simulink model "gazebodemo"  (R2022a)
settings: Solver=FixedStepAuto  StartTime=0.0  StopTime=10.0  FixedStep=0.001  RelTol=1e-3
values from neighbouring files (symbols this model uses):
  alpha = 10000    [Hopf_oscillator_sim.m]    (also in simulation_CPG.m)
  b = 100    [Hopf_oscillator_sim.m]    (also in simulation_CPG.m)
  f1 = 0    [Hopf_oscillator_sim.m]    (also in simulation_CPG.m)
  f2 = 0    [Hopf_oscillator_sim.m]    (also in simulation_CPG.m)
  K_d = diag([500,500])    [simulation_CPG.m]
  K_p = diag([500,500])    [simulation_CPG.m]
  lamda = 1    [Hopf_oscillator_sim.m]    (also in simulation_CPG.m)
  miu = 0.2    [Hopf_oscillator_sim.m]    (also in simulation_CPG.m)
  Tc = 0.001    [simulation_CPG.m]
  wst = (1-beta)/beta*wsw    (= 5.23598775598)    [Hopf_oscillator_sim.m]    (also in simulation_CPG.m)
  wsw = 5*pi    (= 15.7079632679)    [Hopf_oscillator_sim.m]    (also in simulation_CPG.m)
undefined symbols (not defined in the file or in its folder): a, effort, F_v, g, IFV, iner, joint_name, K, LF_body2thigh, LF_thigh2calf, LH_body2thigh, LH_thigh2calf, model_name, pi_m, RF_body2thigh, RF_thigh2calf, RH_body2thigh, RH_thigh2calf
libraries: robotgazebolib x26, simulink x16
settings Model: Creator=liltrump  LastModifiedBy=liltrump

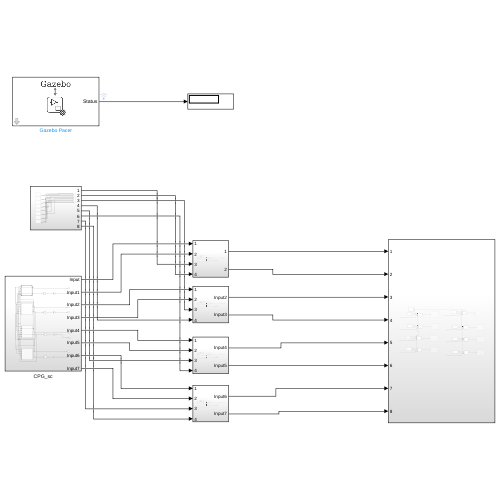
[thumbnail: Simulink's stored preview of the top-level diagram]
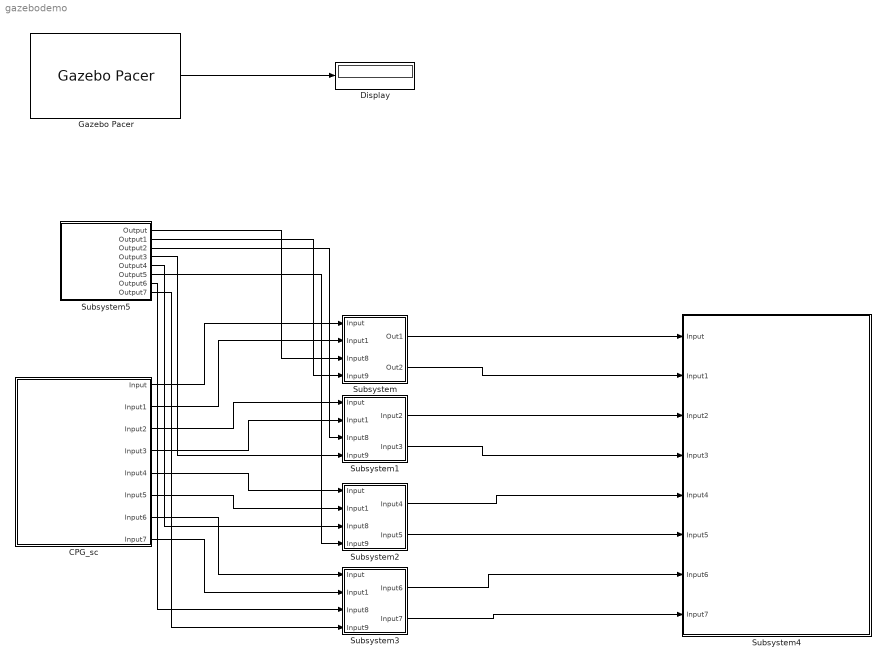
== system gazebodemo ==
  CPG_sc : Subsystem
  Display : Display
  Gazebo Pacer : robotgazebolib/Gazebo Pacer  ResetBehavior=Reset Gazebo simulation time  SampleTime=0.001
      settings: SourceProductBaseCode=RO
  Subsystem : Subsystem
  Subsystem1 : Subsystem
  Subsystem2 : Subsystem
  Subsystem3 : Subsystem
  Subsystem4 : Subsystem
  Subsystem5 : Subsystem
  wires:
  Gazebo Pacer/1 -> Display/1
  CPG_sc/1(Input) -> Subsystem/1(Input)
  CPG_sc/2(Input1) -> Subsystem/2(Input1)
  CPG_sc/3(Input2) -> Subsystem1/1(Input)
  CPG_sc/4(Input3) -> Subsystem1/2(Input1)
  CPG_sc/5(Input4) -> Subsystem2/1(Input)
  CPG_sc/8(Input7) -> Subsystem3/2(Input1)
  CPG_sc/6(Input5) -> Subsystem2/2(Input1)
  CPG_sc/7(Input6) -> Subsystem3/1(Input)
  Subsystem/1(Out1) -> Subsystem4/1(Input)
  Subsystem/2(Out2) -> Subsystem4/2(Input1)
  Subsystem1/1(Input2) -> Subsystem4/3(Input2)
  Subsystem1/2(Input3) -> Subsystem4/4(Input3)
  Subsystem2/1(Input4) -> Subsystem4/5(Input4)
  Subsystem2/2(Input5) -> Subsystem4/6(Input5)
  Subsystem3/1(Input6) -> Subsystem4/7(Input6)
  Subsystem3/2(Input7) -> Subsystem4/8(Input7)
  Subsystem5/1(Output) -> Subsystem/3(Input8)
  Subsystem5/2(Output1) -> Subsystem/4(Input9)
  Subsystem5/3(Output2) -> Subsystem1/3(Input8)
  Subsystem5/4(Output3) -> Subsystem1/4(Input9)
  Subsystem5/5(Output4) -> Subsystem2/3(Input8)
  Subsystem5/6(Output5) -> Subsystem2/4(Input9)
  Subsystem5/7(Output6) -> Subsystem3/3(Input8)
  Subsystem5/8(Output7) -> Subsystem3/4(Input9)

== system gazebodemo/CPG_sc ==
  Gain{,1..3} (4 alike) : Gain  Gain=-2
  Saturation{,1..3} (4 alike) : Saturate  UpperLimit=0  LowerLimit=-1
  Subsystem : Subsystem
  Subsystem1 : Subsystem
  Subsystem2 : Subsystem
  hopf1 : ModelReference  ModelNameDialog=Hopf.slx  SimulationMode=Normal  ModelReferenceVersion=1.13
  Input : Outport
  Input1 : Outport  Port=2
  Input2 : Outport  Port=3
  Input3 : Outport  Port=4
  Input4 : Outport  Port=5
  Input5 : Outport  Port=6
  Input6 : Outport  Port=7
  Input7 : Outport  Port=8
  wires:
  Saturation3/1 -> Gain3/1
  Subsystem2/2(Out2) -> Saturation3/1, Subsystem1/6(In6), Subsystem/6(In6), hopf1/6
  hopf1/1 -> Input/1, Subsystem2/1(In1), Subsystem1/1(In1), Subsystem/1(In1)
  hopf1/2 -> Saturation/1, Subsystem2/2(In2), Subsystem/2(In2), Subsystem1/2(In2)
  Subsystem1/2(Out2) -> Saturation2/1, Subsystem2/6(In6), Subsystem/4(In4), hopf1/4
  Saturation2/1 -> Gain2/1
  Gain/1 -> Input1/1
  Subsystem/2(Out2) -> Saturation1/1, Subsystem2/4(In4), Subsystem1/4(In4), hopf1/2
  Saturation/1 -> Gain/1
  Saturation1/1 -> Gain1/1
  Subsystem/1(Out1) -> Input2/1, Subsystem2/3(In3), Subsystem1/3(In3), hopf1/1
  Subsystem1/1(Out1) -> Input4/1, Subsystem/3(In3), hopf1/3, Subsystem2/5(In5)
  Gain2/1 -> Input5/1
  Subsystem2/1(Out1) -> Input6/1, Subsystem1/5(In5), Subsystem/5(In5), hopf1/5
  Gain1/1 -> Input3/1
  Gain3/1 -> Input7/1

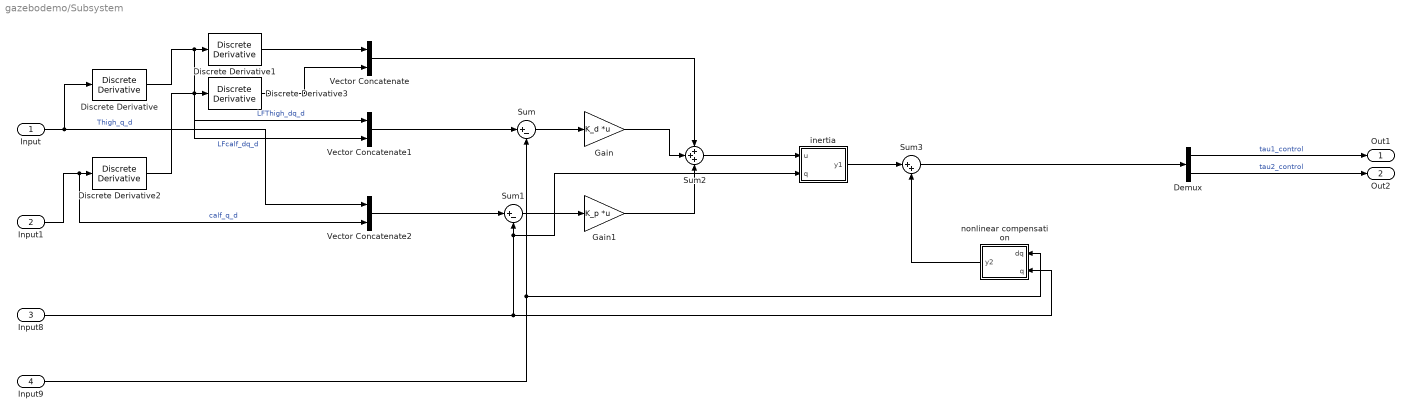
== system gazebodemo/Subsystem ==
  Input : Inport
  Input1 : Inport  Port=2
  Input8 : Inport  Port=3
  Input9 : Inport  Port=4
  Demux : Demux  Outputs=2
  Discrete Derivative{,1..3} (4 alike) : simulink/Discrete/Discrete Derivative  gainval=1.0  ICPrevScaledInput=0.0  OutMin=[]  OutMax=[]  OutDataType=fixdt(1, 16)  OutScaling=2^-10  DoSatur=off
  Gain : Gain  Gain=K_d  Multiplication=Matrix(K*u)
  Gain1 : Gain  Gain=K_p  Multiplication=Matrix(K*u)
  Sum : Sum  Inputs=|+-
  Sum1 : Sum  Inputs=|+-
  Sum2 : Sum  Inputs=+++
  Sum3 : Sum  Inputs=|++
  Vector Concatenate : Concatenate
  Vector Concatenate1 : Concatenate
  Vector Concatenate2 : Concatenate
  inertia : Subsystem
      mask Display: disp('B(q)u')
  nonlinear compensation : Subsystem
      mask Display: disp('n(q,dq)')
  Out1 : Outport
  Out2 : Outport  Port=2
  wires:
  Input/1 -> Vector Concatenate2/1, Discrete Derivative/1  "Thigh_q_d"
  Discrete Derivative/1 -> Vector Concatenate1/1, Discrete Derivative1/1  "LFThigh_dq_d"
  Input1/1 -> Vector Concatenate2/2, Discrete Derivative2/1  "calf_q_d"
  Discrete Derivative2/1 -> Vector Concatenate1/2, Discrete Derivative3/1  "LFcalf_dq_d"
  Gain1/1 -> Sum2/3
  Vector Concatenate1/1 -> Sum/1
  Sum3/1 -> Demux/1
  nonlinear compensation/1(y2) -> Sum3/2
  Vector Concatenate/1 -> Sum2/1
  inertia/1(y1) -> Sum3/1
  Sum/1 -> Gain/1
  Sum2/1 -> inertia/1(u)
  Sum1/1 -> Gain1/1
  Gain/1 -> Sum2/2
  Vector Concatenate2/1 -> Sum1/1
  Discrete Derivative1/1 -> Vector Concatenate/1
  Discrete Derivative3/1 -> Vector Concatenate/2
  Input8/1 -> nonlinear compensation/2(q), inertia/2(q), Sum1/2
  Input9/1 -> Sum/2, nonlinear compensation/1(dq)
  Demux/2 -> Out2/1  "tau2_control"
  Demux/1 -> Out1/1  "tau1_control"

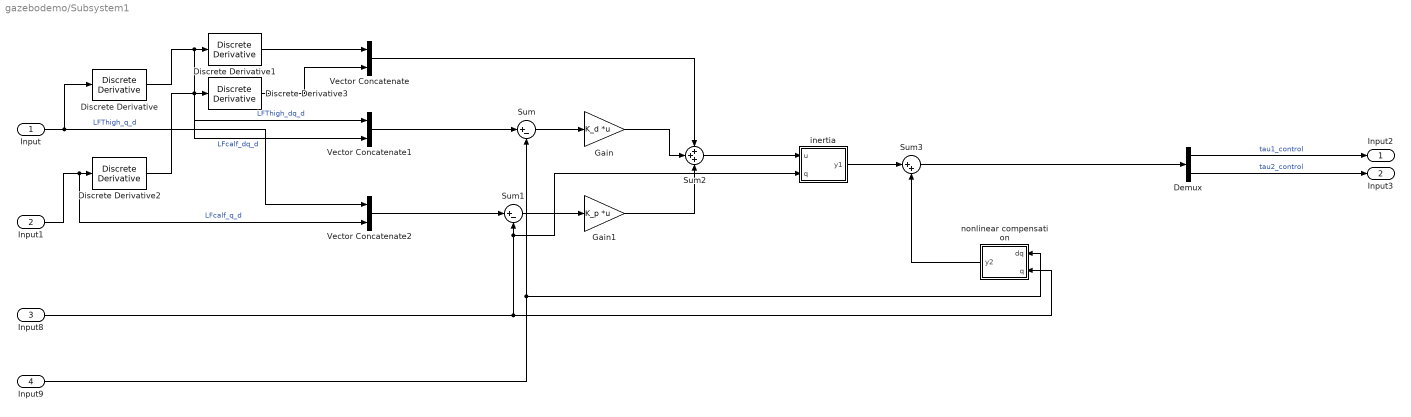
== system gazebodemo/Subsystem1 ==
  Input : Inport
  Input1 : Inport  Port=2
  Input8 : Inport  Port=3
  Input9 : Inport  Port=4
  Demux : Demux  Outputs=2
  Discrete Derivative{,1..3} (4 alike) : simulink/Discrete/Discrete Derivative  gainval=1.0  ICPrevScaledInput=0.0  OutMin=[]  OutMax=[]  OutDataType=fixdt(1, 16)  OutScaling=2^-10  DoSatur=off
  Gain : Gain  Gain=K_d  Multiplication=Matrix(K*u)
  Gain1 : Gain  Gain=K_p  Multiplication=Matrix(K*u)
  Sum : Sum  Inputs=|+-
  Sum1 : Sum  Inputs=|+-
  Sum2 : Sum  Inputs=+++
  Sum3 : Sum  Inputs=|++
  Vector Concatenate : Concatenate
  Vector Concatenate1 : Concatenate
  Vector Concatenate2 : Concatenate
  inertia : Subsystem
      mask Display: disp('B(q)u')
  nonlinear compensation : Subsystem
      mask Display: disp('n(q,dq)')
  Input2 : Outport
  Input3 : Outport  Port=2
  wires:
  Input/1 -> Vector Concatenate2/1, Discrete Derivative/1  "LFThigh_q_d"
  Discrete Derivative/1 -> Vector Concatenate1/1, Discrete Derivative1/1  "LFThigh_dq_d"
  Input1/1 -> Vector Concatenate2/2, Discrete Derivative2/1  "LFcalf_q_d"
  Discrete Derivative2/1 -> Vector Concatenate1/2, Discrete Derivative3/1  "LFcalf_dq_d"
  Gain1/1 -> Sum2/3
  Vector Concatenate1/1 -> Sum/1
  Sum3/1 -> Demux/1
  nonlinear compensation/1(y2) -> Sum3/2
  Vector Concatenate/1 -> Sum2/1
  inertia/1(y1) -> Sum3/1
  Sum/1 -> Gain/1
  Sum2/1 -> inertia/1(u)
  Sum1/1 -> Gain1/1
  Gain/1 -> Sum2/2
  Vector Concatenate2/1 -> Sum1/1
  Discrete Derivative1/1 -> Vector Concatenate/1
  Discrete Derivative3/1 -> Vector Concatenate/2
  Input8/1 -> nonlinear compensation/2(q), inertia/2(q), Sum1/2
  Input9/1 -> Sum/2, nonlinear compensation/1(dq)
  Demux/2 -> Input3/1  "tau2_control"
  Demux/1 -> Input2/1  "tau1_control"

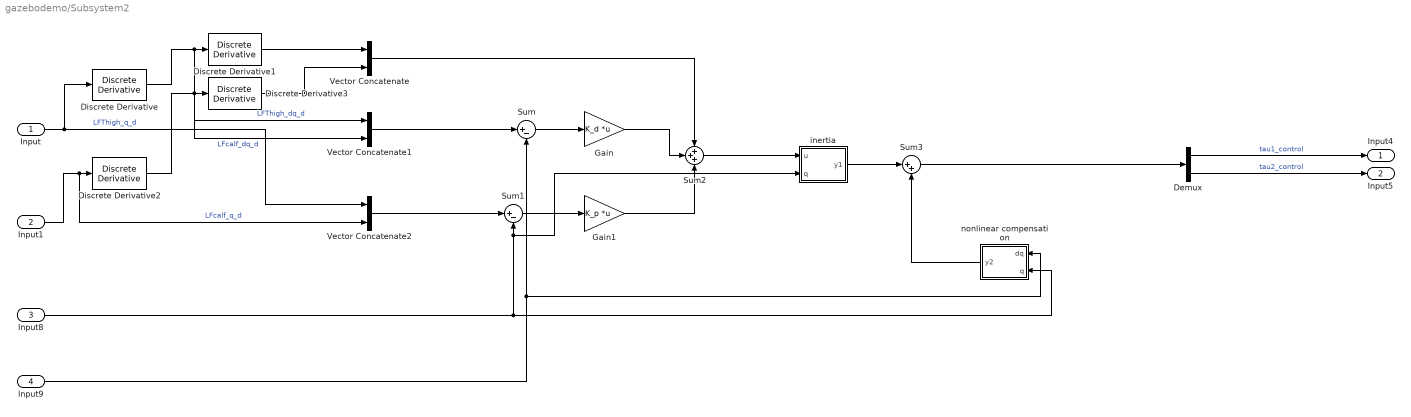
== system gazebodemo/Subsystem2 ==
  Input : Inport
  Input1 : Inport  Port=2
  Input8 : Inport  Port=3
  Input9 : Inport  Port=4
  Demux : Demux  Outputs=2
  Discrete Derivative{,1..3} (4 alike) : simulink/Discrete/Discrete Derivative  gainval=1.0  ICPrevScaledInput=0.0  OutMin=[]  OutMax=[]  OutDataType=fixdt(1, 16)  OutScaling=2^-10  DoSatur=off
  Gain : Gain  Gain=K_d  Multiplication=Matrix(K*u)
  Gain1 : Gain  Gain=K_p  Multiplication=Matrix(K*u)
  Sum : Sum  Inputs=|+-
  Sum1 : Sum  Inputs=|+-
  Sum2 : Sum  Inputs=+++
  Sum3 : Sum  Inputs=|++
  Vector Concatenate : Concatenate
  Vector Concatenate1 : Concatenate
  Vector Concatenate2 : Concatenate
  inertia : Subsystem
      mask Display: disp('B(q)u')
  nonlinear compensation : Subsystem
      mask Display: disp('n(q,dq)')
  Input4 : Outport
  Input5 : Outport  Port=2
  wires:
  Input/1 -> Vector Concatenate2/1, Discrete Derivative/1  "LFThigh_q_d"
  Discrete Derivative/1 -> Vector Concatenate1/1, Discrete Derivative1/1  "LFThigh_dq_d"
  Input1/1 -> Vector Concatenate2/2, Discrete Derivative2/1  "LFcalf_q_d"
  Discrete Derivative2/1 -> Vector Concatenate1/2, Discrete Derivative3/1  "LFcalf_dq_d"
  Gain1/1 -> Sum2/3
  Vector Concatenate1/1 -> Sum/1
  Sum3/1 -> Demux/1
  nonlinear compensation/1(y2) -> Sum3/2
  Vector Concatenate/1 -> Sum2/1
  inertia/1(y1) -> Sum3/1
  Sum/1 -> Gain/1
  Sum2/1 -> inertia/1(u)
  Sum1/1 -> Gain1/1
  Gain/1 -> Sum2/2
  Vector Concatenate2/1 -> Sum1/1
  Discrete Derivative1/1 -> Vector Concatenate/1
  Discrete Derivative3/1 -> Vector Concatenate/2
  Input8/1 -> nonlinear compensation/2(q), inertia/2(q), Sum1/2
  Input9/1 -> Sum/2, nonlinear compensation/1(dq)
  Demux/2 -> Input5/1  "tau2_control"
  Demux/1 -> Input4/1  "tau1_control"

== system gazebodemo/Subsystem3 ==
  Input : Inport
  Input1 : Inport  Port=2
  Input8 : Inport  Port=3
  Input9 : Inport  Port=4
  Demux : Demux  Outputs=2
  Discrete Derivative{,1..3} (4 alike) : simulink/Discrete/Discrete Derivative  gainval=1.0  ICPrevScaledInput=0.0  OutMin=[]  OutMax=[]  OutDataType=fixdt(1, 16)  OutScaling=2^-10  DoSatur=off
  Gain : Gain  Gain=K_d  Multiplication=Matrix(K*u)
  Gain1 : Gain  Gain=K_p  Multiplication=Matrix(K*u)
  Sum : Sum  Inputs=|+-
  Sum1 : Sum  Inputs=|+-
  Sum2 : Sum  Inputs=+++
  Sum3 : Sum  Inputs=|++
  Vector Concatenate : Concatenate
  Vector Concatenate1 : Concatenate
  Vector Concatenate2 : Concatenate
  inertia : Subsystem
      mask Display: disp('B(q)u')
  nonlinear compensation : Subsystem
      mask Display: disp('n(q,dq)')
  Input6 : Outport
  Input7 : Outport  Port=2
  wires:
  Input/1 -> Vector Concatenate2/1, Discrete Derivative/1  "LFThigh_q_d"
  Discrete Derivative/1 -> Vector Concatenate1/1, Discrete Derivative1/1  "LFThigh_dq_d"
  Input1/1 -> Vector Concatenate2/2, Discrete Derivative2/1  "LFcalf_q_d"
  Discrete Derivative2/1 -> Vector Concatenate1/2, Discrete Derivative3/1  "LFcalf_dq_d"
  Gain1/1 -> Sum2/3
  Vector Concatenate1/1 -> Sum/1
  Sum3/1 -> Demux/1
  nonlinear compensation/1(y2) -> Sum3/2
  Vector Concatenate/1 -> Sum2/1
  inertia/1(y1) -> Sum3/1
  Sum/1 -> Gain/1
  Sum2/1 -> inertia/1(u)
  Sum1/1 -> Gain1/1
  Gain/1 -> Sum2/2
  Vector Concatenate2/1 -> Sum1/1
  Discrete Derivative1/1 -> Vector Concatenate/1
  Discrete Derivative3/1 -> Vector Concatenate/2
  Input8/1 -> nonlinear compensation/2(q), inertia/2(q), Sum1/2
  Input9/1 -> Sum/2, nonlinear compensation/1(dq)
  Demux/2 -> Input7/1  "tau2_control"
  Demux/1 -> Input6/1  "tau1_control"

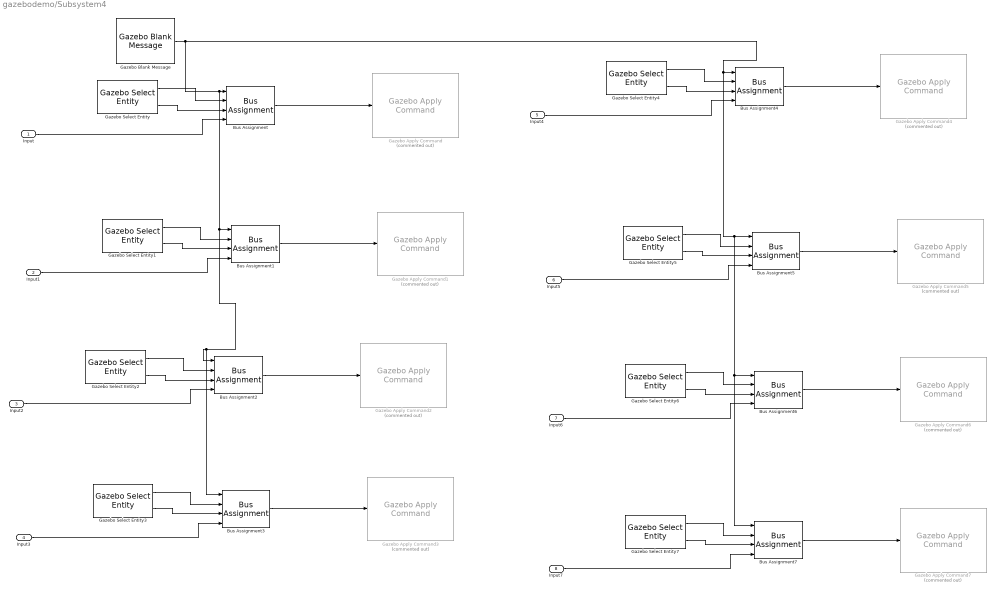
== system gazebodemo/Subsystem4 ==
  Input : Inport
  Input1 : Inport  Port=2
  Input2 : Inport  Port=3
  Input3 : Inport  Port=4
  Input4 : Inport  Port=5
  Input5 : Inport  Port=6
  Input6 : Inport  Port=7
  Input7 : Inport  Port=8
  Bus Assignment{,1..7} (8 alike) : BusAssignment  AssignedSignals=model_name,joint_name,effort
  Gazebo Apply Command{,1..7} (8 alike) : robotgazebolib/Gazebo Apply Command  Commented=on  cmdType=ApplyJointTorque  sampleTime=0.001
      settings: SourceProductBaseCode=RO
  Gazebo Blank Message : robotgazebolib/Gazebo Blank Message  msgType=ApplyJointTorque  sampleTime=0.001  busName='Gazebo_SL_Bus_gazebo_msgs_ApplyJointTorque'
      settings: SourceProductBaseCode=RO
  Gazebo Select Entity : robotgazebolib/Gazebo Select Entity  modelElemName=IFV/LF_body2thigh  outputArraySize=128  OutputLabel=Joint  SelectType=Joint
      settings: SourceProductBaseCode=RO
  Gazebo Select Entity1 : robotgazebolib/Gazebo Select Entity  modelElemName=IFV/LF_thigh2calf  outputArraySize=128  OutputLabel=Joint  SelectType=Joint
      settings: SourceProductBaseCode=RO
  Gazebo Select Entity2 : robotgazebolib/Gazebo Select Entity  modelElemName=IFV/RF_body2thigh  outputArraySize=128  OutputLabel=Joint  SelectType=Joint
      settings: SourceProductBaseCode=RO
  Gazebo Select Entity3 : robotgazebolib/Gazebo Select Entity  modelElemName=IFV/RF_thigh2calf  outputArraySize=128  OutputLabel=Joint  SelectType=Joint
      settings: SourceProductBaseCode=RO
  Gazebo Select Entity4 : robotgazebolib/Gazebo Select Entity  modelElemName=IFV/LH_body2thigh  outputArraySize=128  OutputLabel=Joint  SelectType=Joint
      settings: SourceProductBaseCode=RO
  Gazebo Select Entity5 : robotgazebolib/Gazebo Select Entity  modelElemName=IFV/LH_thigh2calf  outputArraySize=128  OutputLabel=Joint  SelectType=Joint
      settings: SourceProductBaseCode=RO
  Gazebo Select Entity6 : robotgazebolib/Gazebo Select Entity  modelElemName=IFV/RH_body2thigh  outputArraySize=128  OutputLabel=Joint  SelectType=Joint
      settings: SourceProductBaseCode=RO
  Gazebo Select Entity7 : robotgazebolib/Gazebo Select Entity  modelElemName=IFV/RH_thigh2calf  outputArraySize=128  OutputLabel=Joint  SelectType=Joint
      settings: SourceProductBaseCode=RO
  wires:
  Gazebo Select Entity/1 -> Bus Assignment/2
  Gazebo Select Entity/2 -> Bus Assignment/3
  Bus Assignment/1 -> Gazebo Apply Command/1
  Input/1 -> Bus Assignment/4
  Bus Assignment1/1 -> Gazebo Apply Command1/1
  Input1/1 -> Bus Assignment1/4
  Gazebo Select Entity1/1 -> Bus Assignment1/2
  Gazebo Select Entity1/2 -> Bus Assignment1/3
  Bus Assignment2/1 -> Gazebo Apply Command2/1
  Input2/1 -> Bus Assignment2/4
  Gazebo Select Entity2/1 -> Bus Assignment2/2
  Gazebo Select Entity2/2 -> Bus Assignment2/3
  Bus Assignment3/1 -> Gazebo Apply Command3/1
  Input3/1 -> Bus Assignment3/4
  Gazebo Select Entity3/1 -> Bus Assignment3/2
  Gazebo Select Entity3/2 -> Bus Assignment3/3
  Bus Assignment4/1 -> Gazebo Apply Command4/1
  Input4/1 -> Bus Assignment4/4
  Gazebo Select Entity4/1 -> Bus Assignment4/2
  Gazebo Select Entity4/2 -> Bus Assignment4/3
  Bus Assignment5/1 -> Gazebo Apply Command5/1
  Input5/1 -> Bus Assignment5/4
  Gazebo Select Entity5/1 -> Bus Assignment5/2
  Gazebo Select Entity5/2 -> Bus Assignment5/3
  Bus Assignment6/1 -> Gazebo Apply Command6/1
  Input6/1 -> Bus Assignment6/4
  Gazebo Select Entity6/1 -> Bus Assignment6/2
  Gazebo Select Entity6/2 -> Bus Assignment6/3
  Bus Assignment7/1 -> Gazebo Apply Command7/1
  Input7/1 -> Bus Assignment7/4
  Gazebo Select Entity7/1 -> Bus Assignment7/2
  Gazebo Blank Message/1 -> Bus Assignment7/1, Bus Assignment6/1, Bus Assignment5/1, Bus Assignment4/1, Bus Assignment3/1, Bus Assignment2/1, Bus Assignment1/1, Bus Assignment/1
  Gazebo Select Entity7/2 -> Bus Assignment7/3

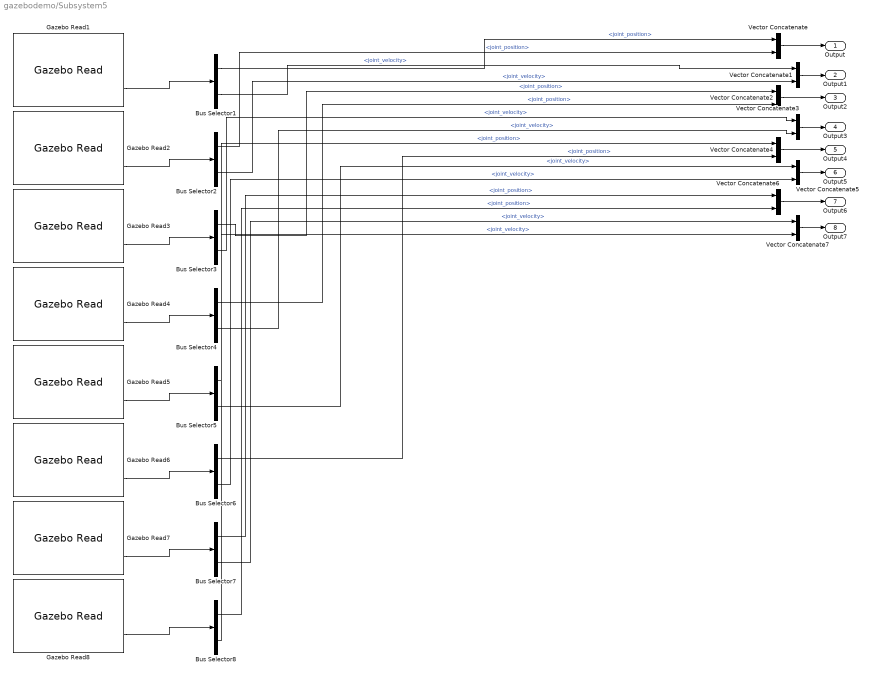
== system gazebodemo/Subsystem5 ==
  Bus Selector{1..8} (8 alike) : BusSelector  OutputSignals=joint_position,joint_velocity
  Gazebo Read1 : robotgazebolib/Gazebo Read  topicSource=From Gazebo  topic=/gazebo/ground_truth/joint_state/IFV/LF_body2thigh  messageType=gazebo_msgs/JointState  sampleTime=0.001
      settings: SourceProductBaseCode=RO
  Gazebo Read2 : robotgazebolib/Gazebo Read  topicSource=From Gazebo  topic=/gazebo/ground_truth/joint_state/IFV/LF_thigh2calf  messageType=gazebo_msgs/JointState  sampleTime=0.001
      settings: SourceProductBaseCode=RO
  Gazebo Read3 : robotgazebolib/Gazebo Read  topicSource=From Gazebo  topic=/gazebo/ground_truth/joint_state/IFV/RF_body2thigh  messageType=gazebo_msgs/JointState  sampleTime=0.001
      settings: SourceProductBaseCode=RO
  Gazebo Read4 : robotgazebolib/Gazebo Read  topicSource=From Gazebo  topic=/gazebo/ground_truth/joint_state/IFV/RF_thigh2calf  messageType=gazebo_msgs/JointState  sampleTime=0.001
      settings: SourceProductBaseCode=RO
  Gazebo Read5 : robotgazebolib/Gazebo Read  topicSource=From Gazebo  topic=/gazebo/ground_truth/joint_state/IFV/LH_body2thigh  messageType=gazebo_msgs/JointState  sampleTime=0.001
      settings: SourceProductBaseCode=RO
  Gazebo Read6 : robotgazebolib/Gazebo Read  topicSource=From Gazebo  topic=/gazebo/ground_truth/joint_state/IFV/LF_thigh2calf  messageType=gazebo_msgs/JointState  sampleTime=0.001
      settings: SourceProductBaseCode=RO
  Gazebo Read7 : robotgazebolib/Gazebo Read  topicSource=From Gazebo  topic=/gazebo/ground_truth/joint_state/IFV/RH_body2thigh  messageType=gazebo_msgs/JointState  sampleTime=0.001
      settings: SourceProductBaseCode=RO
  Gazebo Read8 : robotgazebolib/Gazebo Read  topicSource=From Gazebo  topic=/gazebo/ground_truth/joint_state/IFV/RH_thigh2calf  messageType=gazebo_msgs/JointState  sampleTime=0.001
      settings: SourceProductBaseCode=RO
  Vector Concatenate{,1..7} (8 alike) : Concatenate
  Output : Outport
  Output1 : Outport  Port=2
  Output2 : Outport  Port=3
  Output3 : Outport  Port=4
  Output4 : Outport  Port=5
  Output5 : Outport  Port=6
  Output6 : Outport  Port=7
  Output7 : Outport  Port=8
  wires:
  Gazebo Read1/2 -> Bus Selector1/1
  Bus Selector1/2 -> Vector Concatenate1/1  "<joint_velocity>"
  Bus Selector1/1 -> Vector Concatenate/1  "<joint_position>"
  Bus Selector2/2 -> Vector Concatenate1/2  "<joint_velocity>"
  Gazebo Read2/2 -> Bus Selector2/1
  Bus Selector2/1 -> Vector Concatenate/2  "<joint_position>"
  Bus Selector3/2 -> Vector Concatenate3/1  "<joint_velocity>"
  Gazebo Read3/2 -> Bus Selector3/1
  Bus Selector3/1 -> Vector Concatenate2/1  "<joint_position>"
  Bus Selector4/2 -> Vector Concatenate3/2  "<joint_velocity>"
  Gazebo Read4/2 -> Bus Selector4/1
  Bus Selector4/1 -> Vector Concatenate2/2  "<joint_position>"
  Bus Selector5/2 -> Vector Concatenate5/1  "<joint_velocity>"
  Gazebo Read5/2 -> Bus Selector5/1
  Bus Selector5/1 -> Vector Concatenate4/1  "<joint_position>"
  Bus Selector6/2 -> Vector Concatenate5/2  "<joint_velocity>"
  Gazebo Read6/2 -> Bus Selector6/1
  Bus Selector6/1 -> Vector Concatenate4/2  "<joint_position>"
  Bus Selector7/2 -> Vector Concatenate7/1  "<joint_velocity>"
  Gazebo Read7/2 -> Bus Selector7/1
  Bus Selector7/1 -> Vector Concatenate6/1  "<joint_position>"
  Bus Selector8/2 -> Vector Concatenate7/2  "<joint_velocity>"
  Gazebo Read8/2 -> Bus Selector8/1
  Bus Selector8/1 -> Vector Concatenate6/2  "<joint_position>"
  Vector Concatenate/1 -> Output/1
  Vector Concatenate1/1 -> Output1/1
  Vector Concatenate2/1 -> Output2/1
  Vector Concatenate3/1 -> Output3/1
  Vector Concatenate4/1 -> Output4/1
  Vector Concatenate5/1 -> Output5/1
  Vector Concatenate6/1 -> Output6/1
  Vector Concatenate7/1 -> Output7/1

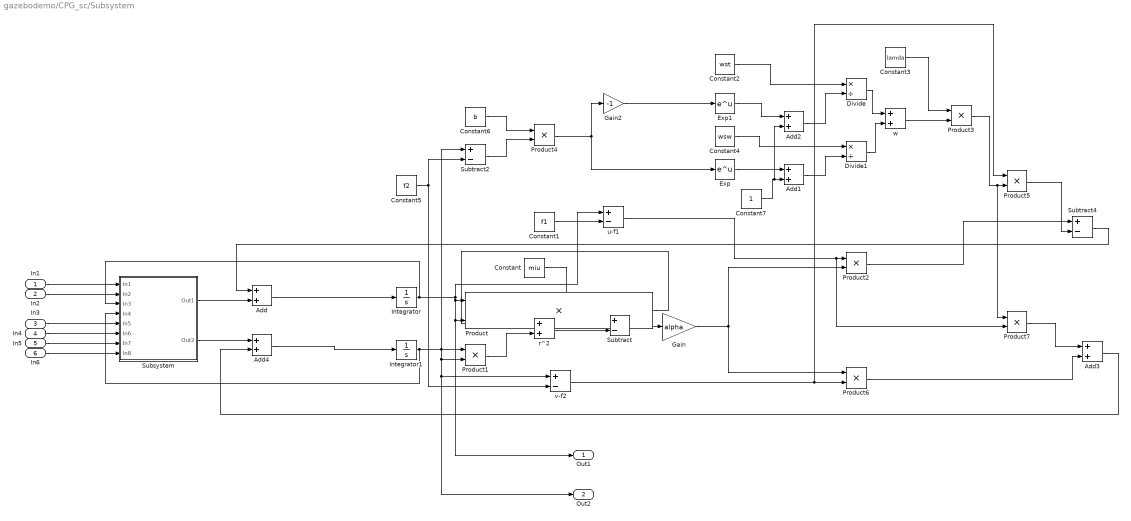
== system gazebodemo/CPG_sc/Subsystem ==
  In1 : Inport
  In2 : Inport  Port=2
  In3 : Inport  Port=3
  In4 : Inport  Port=4
  In5 : Inport  Port=5
  In6 : Inport  Port=6
  Add{,1..4} (5 alike) : Sum
  Constant : Constant  Value=miu
  Constant1 : Constant  Value=f1
  Constant2 : Constant  Value=wst
  Constant3 : Constant  Value=lamda
  Constant4 : Constant  Value=wsw
  Constant5 : Constant  Value=f2
  Constant6 : Constant  Value=b
  Constant7 : Constant
  Divide : Product  Inputs=*/
  Divide1 : Product  Inputs=*/
  Exp : Math
  Exp1 : Math
  Gain : Gain  Gain=alpha
  Gain2 : Gain  Gain=-1
  Integrator : Integrator
  Integrator1 : Integrator
  Product{,1..7} (8 alike) : Product
  Subsystem : Subsystem
  Subtract : Sum  Inputs=+-
  Subtract2 : Sum  Inputs=+-
  Subtract4 : Sum  Inputs=+-
  r^2 : Sum
  u-f1 : Sum  Inputs=+-
  v-f2 : Sum  Inputs=+-
  w : Sum
  Out1 : Outport
  Out2 : Outport  Port=2
  wires:
  Constant2/1 -> Divide/1
  Exp1/1 -> Add2/1
  w/1 -> Product3/2
  Subsystem/2(Out2) -> Add4/1
  Subtract4/1 -> Add/1
  Constant/1 -> Subtract/1
  Add4/1 -> Integrator1/1
  r^2/1 -> Subtract/2
  Gain/1 -> Product6/1, Product2/2
  v-f2/1 -> Product5/1, Product6/2
  Add1/1 -> Divide1/2
  Subsystem/1(Out1) -> Add/2
  Add3/1 -> Add4/2
  Product7/1 -> Add3/1
  Constant1/1 -> u-f1/2
  Exp/1 -> Add1/1
  Product6/1 -> Add3/2
  Divide1/1 -> w/2
  Constant6/1 -> Product4/1
  u-f1/1 -> Product7/2, Product2/1
  Constant5/1 -> v-f2/2, Subtract2/2
  Constant4/1 -> Divide1/1
  Product3/1 -> Product7/1, Product5/2
  Divide/1 -> w/1
  Gain2/1 -> Exp1/1
  Add/1 -> Integrator/1
  Add2/1 -> Divide/2
  Constant3/1 -> Product3/1
  Product4/1 -> Exp/1, Gain2/1
  Subtract2/1 -> Product4/2
  Product1/1 -> r^2/2
  Product/1 -> r^2/1
  Integrator1/1 -> Subsystem/4(In4), Out2/1, v-f2/1, Product1/2, Product1/1, Subtract2/1
  Integrator/1 -> Subsystem/3(In3), Product/2, Out1/1, Product/1, u-f1/1
  Product5/1 -> Subtract4/2
  In1/1 -> Subsystem/1(In1)
  Product2/1 -> Subtract4/1
  In2/1 -> Subsystem/2(In2)
  Subtract/1 -> Gain/1
  In3/1 -> Subsystem/5(In5)
  In5/1 -> Subsystem/7(In7)
  In6/1 -> Subsystem/8(In8)
  Constant7/1 -> Add2/2, Add1/2
  In4/1 -> Subsystem/6(In6)

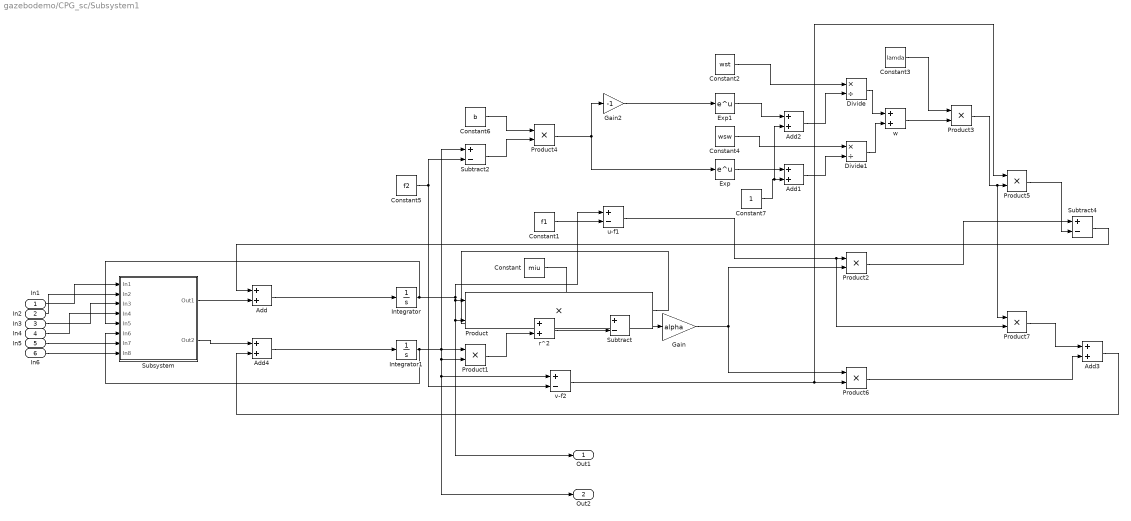
== system gazebodemo/CPG_sc/Subsystem1 ==
  In1 : Inport
  In2 : Inport  Port=2
  In3 : Inport  Port=3
  In4 : Inport  Port=4
  In5 : Inport  Port=5
  In6 : Inport  Port=6
  Add{,1..4} (5 alike) : Sum
  Constant : Constant  Value=miu
  Constant1 : Constant  Value=f1
  Constant2 : Constant  Value=wst
  Constant3 : Constant  Value=lamda
  Constant4 : Constant  Value=wsw
  Constant5 : Constant  Value=f2
  Constant6 : Constant  Value=b
  Constant7 : Constant
  Divide : Product  Inputs=*/
  Divide1 : Product  Inputs=*/
  Exp : Math
  Exp1 : Math
  Gain : Gain  Gain=alpha
  Gain2 : Gain  Gain=-1
  Integrator : Integrator
  Integrator1 : Integrator
  Product{,1..7} (8 alike) : Product
  Subsystem : Subsystem
  Subtract : Sum  Inputs=+-
  Subtract2 : Sum  Inputs=+-
  Subtract4 : Sum  Inputs=+-
  r^2 : Sum
  u-f1 : Sum  Inputs=+-
  v-f2 : Sum  Inputs=+-
  w : Sum
  Out1 : Outport
  Out2 : Outport  Port=2
  wires:
  Constant2/1 -> Divide/1
  Exp1/1 -> Add2/1
  w/1 -> Product3/2
  Subsystem/2(Out2) -> Add4/1
  Subtract4/1 -> Add/1
  Constant/1 -> Subtract/1
  Add4/1 -> Integrator1/1
  r^2/1 -> Subtract/2
  Gain/1 -> Product6/1, Product2/2
  v-f2/1 -> Product5/1, Product6/2
  Add1/1 -> Divide1/2
  Subsystem/1(Out1) -> Add/2
  Add3/1 -> Add4/2
  Product7/1 -> Add3/1
  Constant1/1 -> u-f1/2
  Exp/1 -> Add1/1
  Product6/1 -> Add3/2
  Divide1/1 -> w/2
  Constant6/1 -> Product4/1
  u-f1/1 -> Product7/2, Product2/1
  Constant5/1 -> v-f2/2, Subtract2/2
  Constant4/1 -> Divide1/1
  Product3/1 -> Product7/1, Product5/2
  Divide/1 -> w/1
  Gain2/1 -> Exp1/1
  Add/1 -> Integrator/1
  Add2/1 -> Divide/2
  Constant3/1 -> Product3/1
  Product4/1 -> Exp/1, Gain2/1
  Subtract2/1 -> Product4/2
  Product1/1 -> r^2/2
  Product/1 -> r^2/1
  Integrator1/1 -> Subsystem/6(In6), Out2/1, v-f2/1, Product1/2, Product1/1, Subtract2/1
  Integrator/1 -> Subsystem/5(In5), Product/2, Out1/1, Product/1, u-f1/1
  Product5/1 -> Subtract4/2
  In1/1 -> Subsystem/1(In1)
  Product2/1 -> Subtract4/1
  In2/1 -> Subsystem/2(In2)
  Subtract/1 -> Gain/1
  In5/1 -> Subsystem/7(In7)
  In6/1 -> Subsystem/8(In8)
  Constant7/1 -> Add2/2, Add1/2
  In3/1 -> Subsystem/3(In3)
  In4/1 -> Subsystem/4(In4)

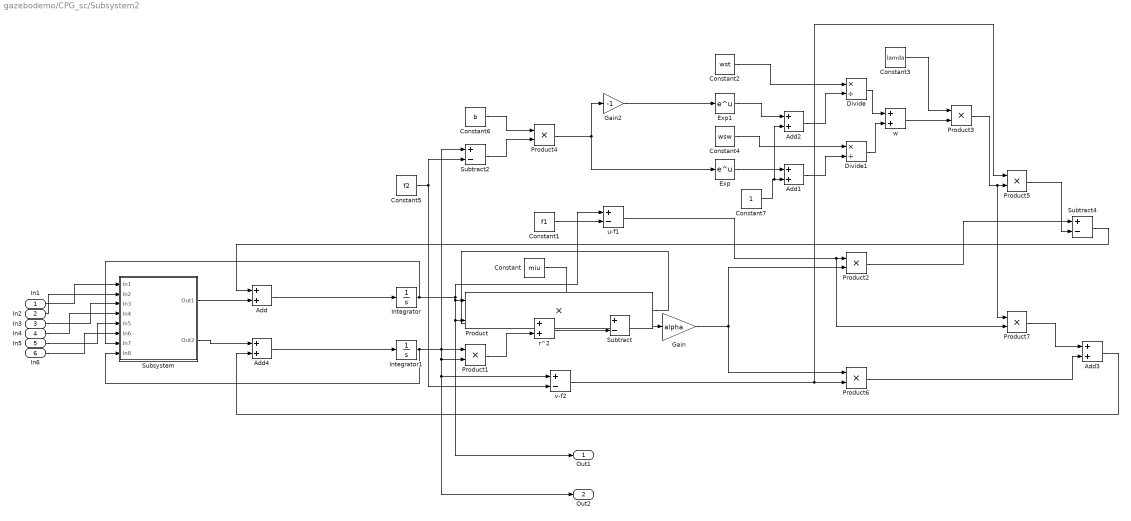
== system gazebodemo/CPG_sc/Subsystem2 ==
  In1 : Inport
  In2 : Inport  Port=2
  In3 : Inport  Port=3
  In4 : Inport  Port=4
  In5 : Inport  Port=5
  In6 : Inport  Port=6
  Add{,1..4} (5 alike) : Sum
  Constant : Constant  Value=miu
  Constant1 : Constant  Value=f1
  Constant2 : Constant  Value=wst
  Constant3 : Constant  Value=lamda
  Constant4 : Constant  Value=wsw
  Constant5 : Constant  Value=f2
  Constant6 : Constant  Value=b
  Constant7 : Constant
  Divide : Product  Inputs=*/
  Divide1 : Product  Inputs=*/
  Exp : Math
  Exp1 : Math
  Gain : Gain  Gain=alpha
  Gain2 : Gain  Gain=-1
  Integrator : Integrator
  Integrator1 : Integrator
  Product{,1..7} (8 alike) : Product
  Subsystem : Subsystem
  Subtract : Sum  Inputs=+-
  Subtract2 : Sum  Inputs=+-
  Subtract4 : Sum  Inputs=+-
  r^2 : Sum
  u-f1 : Sum  Inputs=+-
  v-f2 : Sum  Inputs=+-
  w : Sum
  Out1 : Outport
  Out2 : Outport  Port=2
  wires:
  Constant2/1 -> Divide/1
  Exp1/1 -> Add2/1
  w/1 -> Product3/2
  Subsystem/2(Out2) -> Add4/1
  Subtract4/1 -> Add/1
  Constant/1 -> Subtract/1
  Add4/1 -> Integrator1/1
  r^2/1 -> Subtract/2
  Gain/1 -> Product6/1, Product2/2
  v-f2/1 -> Product5/1, Product6/2
  Add1/1 -> Divide1/2
  Subsystem/1(Out1) -> Add/2
  Add3/1 -> Add4/2
  Product7/1 -> Add3/1
  Constant1/1 -> u-f1/2
  Exp/1 -> Add1/1
  Product6/1 -> Add3/2
  Divide1/1 -> w/2
  Constant6/1 -> Product4/1
  u-f1/1 -> Product7/2, Product2/1
  Constant5/1 -> v-f2/2, Subtract2/2
  Constant4/1 -> Divide1/1
  Product3/1 -> Product7/1, Product5/2
  Divide/1 -> w/1
  Gain2/1 -> Exp1/1
  Add/1 -> Integrator/1
  Add2/1 -> Divide/2
  Constant3/1 -> Product3/1
  Product4/1 -> Exp/1, Gain2/1
  Subtract2/1 -> Product4/2
  Product1/1 -> r^2/2
  Product/1 -> r^2/1
  Integrator1/1 -> Subsystem/8(In8), Out2/1, v-f2/1, Product1/2, Product1/1, Subtract2/1
  Integrator/1 -> Subsystem/7(In7), Product/2, Out1/1, Product/1, u-f1/1
  Product5/1 -> Subtract4/2
  In1/1 -> Subsystem/1(In1)
  Product2/1 -> Subtract4/1
  In2/1 -> Subsystem/2(In2)
  Subtract/1 -> Gain/1
  Constant7/1 -> Add2/2, Add1/2
  In3/1 -> Subsystem/3(In3)
  In4/1 -> Subsystem/4(In4)
  In5/1 -> Subsystem/5(In5)
  In6/1 -> Subsystem/6(In6)

== system gazebodemo/Subsystem/inertia ==
  u : Inport
  q : Inport  Port=2
  Fcn : Fcn  Expr=cos(u(2))  SampleTime=Tc
  Mux : Mux  Inputs=[2,1]
  "invB " : MATLABFcn  MATLABFcn=iner(u(3))*u(1:2)  OutputDimensions=2  SampleTime=Tc
      mask Display: disp('B(q)')
  y1 : Outport  InitialOutput=0
  wires:
  u/1 -> Mux/1
  q/1 -> Fcn/1
  Mux/1 -> "invB "/1
  "invB "/1 -> y1/1
  Fcn/1 -> Mux/2

== system gazebodemo/Subsystem/nonlinear compensation ==
  dq : Inport
  q : Inport  Port=2
  Coriolis + centrifugal : Subsystem
      mask Display: disp('C(q,dq)dq')
  Sum4 : Sum  Inputs=+++  InputSameDT=on  SaturateOnIntegerOverflow=on  OutDataTypeStr=Inherit: Same as first input
  friction : Gain  Gain=F_v  Multiplication=Matrix(K*u)  SaturateOnIntegerOverflow=on  SampleTime=Tc  OutDataTypeStr=Inherit: Same as input  ParamDataTypeStr=Inherit: Same as input
      mask Display: disp('F_v')
  gravity : Subsystem
      mask Display: disp('g(q)')
  y2 : Outport  InitialOutput=0
  wires:
  Coriolis + centrifugal/1(Cdq) -> Sum4/2
  dq/1 -> friction/1, Coriolis + centrifugal/2(dq)
  q/1 -> Coriolis + centrifugal/1(q), gravity/1(q)
  friction/1 -> Sum4/3
  Sum4/1 -> y2/1
  gravity/1(g) -> Sum4/1

== system gazebodemo/Subsystem1/inertia ==
  u : Inport
  q : Inport  Port=2
  Fcn : Fcn  Expr=cos(u(2))  SampleTime=Tc
  Mux : Mux  Inputs=[2,1]
  "invB " : MATLABFcn  MATLABFcn=iner(u(3))*u(1:2)  OutputDimensions=2  SampleTime=Tc
      mask Display: disp('B(q)')
  y1 : Outport  InitialOutput=0
  wires:
  u/1 -> Mux/1
  q/1 -> Fcn/1
  Mux/1 -> "invB "/1
  "invB "/1 -> y1/1
  Fcn/1 -> Mux/2

== system gazebodemo/Subsystem1/nonlinear compensation ==
  dq : Inport
  q : Inport  Port=2
  Coriolis + centrifugal : Subsystem
      mask Display: disp('C(q,dq)dq')
  Sum4 : Sum  Inputs=+++  InputSameDT=on  SaturateOnIntegerOverflow=on  OutDataTypeStr=Inherit: Same as first input
  friction : Gain  Gain=F_v  Multiplication=Matrix(K*u)  SaturateOnIntegerOverflow=on  SampleTime=Tc  OutDataTypeStr=Inherit: Same as input  ParamDataTypeStr=Inherit: Same as input
      mask Display: disp('F_v')
  gravity : Subsystem
      mask Display: disp('g(q)')
  y2 : Outport  InitialOutput=0
  wires:
  Coriolis + centrifugal/1(Cdq) -> Sum4/2
  dq/1 -> friction/1, Coriolis + centrifugal/2(dq)
  q/1 -> Coriolis + centrifugal/1(q), gravity/1(q)
  friction/1 -> Sum4/3
  Sum4/1 -> y2/1
  gravity/1(g) -> Sum4/1

== system gazebodemo/Subsystem2/inertia ==
  u : Inport
  q : Inport  Port=2
  Fcn : Fcn  Expr=cos(u(2))  SampleTime=Tc
  Mux : Mux  Inputs=[2,1]
  "invB " : MATLABFcn  MATLABFcn=iner(u(3))*u(1:2)  OutputDimensions=2  SampleTime=Tc
      mask Display: disp('B(q)')
  y1 : Outport  InitialOutput=0
  wires:
  u/1 -> Mux/1
  q/1 -> Fcn/1
  Mux/1 -> "invB "/1
  "invB "/1 -> y1/1
  Fcn/1 -> Mux/2

== system gazebodemo/Subsystem2/nonlinear compensation ==
  dq : Inport
  q : Inport  Port=2
  Coriolis + centrifugal : Subsystem
      mask Display: disp('C(q,dq)dq')
  Sum4 : Sum  Inputs=+++  InputSameDT=on  SaturateOnIntegerOverflow=on  OutDataTypeStr=Inherit: Same as first input
  friction : Gain  Gain=F_v  Multiplication=Matrix(K*u)  SaturateOnIntegerOverflow=on  SampleTime=Tc  OutDataTypeStr=Inherit: Same as input  ParamDataTypeStr=Inherit: Same as input
      mask Display: disp('F_v')
  gravity : Subsystem
      mask Display: disp('g(q)')
  y2 : Outport  InitialOutput=0
  wires:
  Coriolis + centrifugal/1(Cdq) -> Sum4/2
  dq/1 -> friction/1, Coriolis + centrifugal/2(dq)
  q/1 -> Coriolis + centrifugal/1(q), gravity/1(q)
  friction/1 -> Sum4/3
  Sum4/1 -> y2/1
  gravity/1(g) -> Sum4/1

== system gazebodemo/Subsystem3/inertia ==
  u : Inport
  q : Inport  Port=2
  Fcn : Fcn  Expr=cos(u(2))  SampleTime=Tc
  Mux : Mux  Inputs=[2,1]
  "invB " : MATLABFcn  MATLABFcn=iner(u(3))*u(1:2)  OutputDimensions=2  SampleTime=Tc
      mask Display: disp('B(q)')
  y1 : Outport  InitialOutput=0
  wires:
  u/1 -> Mux/1
  q/1 -> Fcn/1
  Mux/1 -> "invB "/1
  "invB "/1 -> y1/1
  Fcn/1 -> Mux/2

== system gazebodemo/Subsystem3/nonlinear compensation ==
  dq : Inport
  q : Inport  Port=2
  Coriolis + centrifugal : Subsystem
      mask Display: disp('C(q,dq)dq')
  Sum4 : Sum  Inputs=+++  InputSameDT=on  SaturateOnIntegerOverflow=on  OutDataTypeStr=Inherit: Same as first input
  friction : Gain  Gain=F_v  Multiplication=Matrix(K*u)  SaturateOnIntegerOverflow=on  SampleTime=Tc  OutDataTypeStr=Inherit: Same as input  ParamDataTypeStr=Inherit: Same as input
      mask Display: disp('F_v')
  gravity : Subsystem
      mask Display: disp('g(q)')
  y2 : Outport  InitialOutput=0
  wires:
  Coriolis + centrifugal/1(Cdq) -> Sum4/2
  dq/1 -> friction/1, Coriolis + centrifugal/2(dq)
  q/1 -> Coriolis + centrifugal/1(q), gravity/1(q)
  friction/1 -> Sum4/3
  Sum4/1 -> y2/1
  gravity/1(g) -> Sum4/1

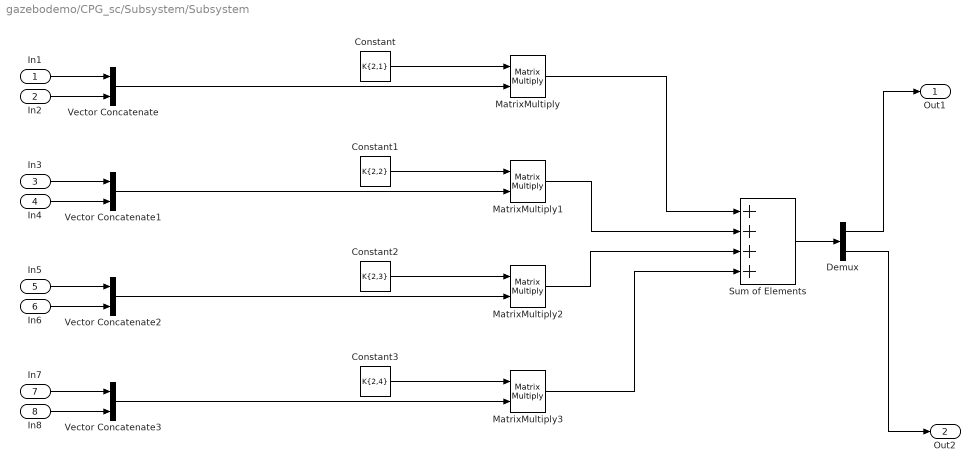
== system gazebodemo/CPG_sc/Subsystem/Subsystem ==
  In1 : Inport
  In2 : Inport  Port=2
  In3 : Inport  Port=3
  In4 : Inport  Port=4
  In5 : Inport  Port=5
  In6 : Inport  Port=6
  In7 : Inport  Port=7
  In8 : Inport  Port=8
  Constant : Constant  Value=K{2,1}  VectorParams1D=off
  Constant1 : Constant  Value=K{2,2}  VectorParams1D=off
  Constant2 : Constant  Value=K{2,3}  VectorParams1D=off
  Constant3 : Constant  Value=K{2,4}  VectorParams1D=off
  Demux : Demux  Outputs=2
  MatrixMultiply{,1..3} (4 alike) : Product  Multiplication=Matrix(*)
  Sum of Elements : Sum  Inputs=++++
  Vector Concatenate{,1..3} (4 alike) : Concatenate
  Out1 : Outport
  Out2 : Outport  Port=2
  wires:
  In1/1 -> Vector Concatenate/1
  In2/1 -> Vector Concatenate/2
  Vector Concatenate/1 -> MatrixMultiply/2
  Constant/1 -> MatrixMultiply/1
  Constant1/1 -> MatrixMultiply1/1
  Constant2/1 -> MatrixMultiply2/1
  Constant3/1 -> MatrixMultiply3/1
  MatrixMultiply/1 -> Sum of Elements/1
  MatrixMultiply1/1 -> Sum of Elements/2
  MatrixMultiply2/1 -> Sum of Elements/3
  MatrixMultiply3/1 -> Sum of Elements/4
  Sum of Elements/1 -> Demux/1
  Demux/1 -> Out1/1
  Demux/2 -> Out2/1
  In4/1 -> Vector Concatenate1/2
  In5/1 -> Vector Concatenate2/1
  In6/1 -> Vector Concatenate2/2
  In7/1 -> Vector Concatenate3/1
  In8/1 -> Vector Concatenate3/2
  Vector Concatenate1/1 -> MatrixMultiply1/2
  Vector Concatenate2/1 -> MatrixMultiply2/2
  Vector Concatenate3/1 -> MatrixMultiply3/2
  In3/1 -> Vector Concatenate1/1

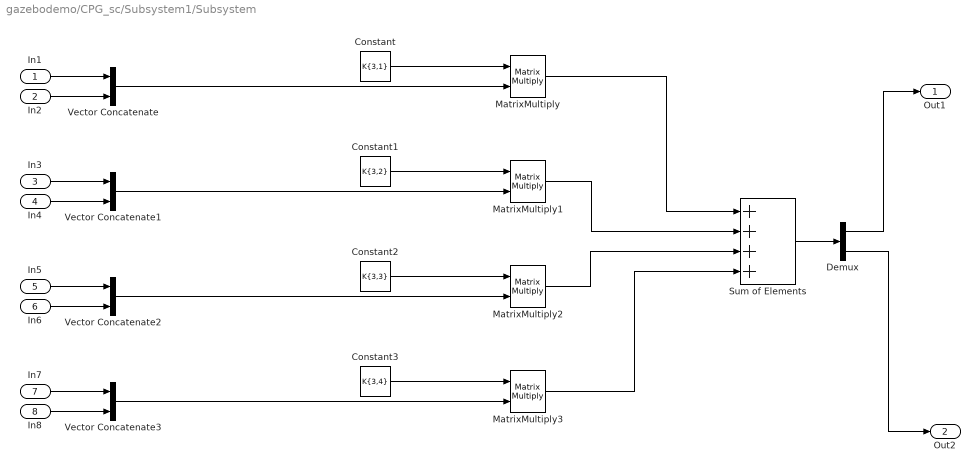
== system gazebodemo/CPG_sc/Subsystem1/Subsystem ==
  In1 : Inport
  In2 : Inport  Port=2
  In3 : Inport  Port=3
  In4 : Inport  Port=4
  In5 : Inport  Port=5
  In6 : Inport  Port=6
  In7 : Inport  Port=7
  In8 : Inport  Port=8
  Constant : Constant  Value=K{3,1}  VectorParams1D=off
  Constant1 : Constant  Value=K{3,2}  VectorParams1D=off
  Constant2 : Constant  Value=K{3,3}  VectorParams1D=off
  Constant3 : Constant  Value=K{3,4}  VectorParams1D=off
  Demux : Demux  Outputs=2
  MatrixMultiply{,1..3} (4 alike) : Product  Multiplication=Matrix(*)
  Sum of Elements : Sum  Inputs=++++
  Vector Concatenate{,1..3} (4 alike) : Concatenate
  Out1 : Outport
  Out2 : Outport  Port=2
  wires:
  In1/1 -> Vector Concatenate/1
  In2/1 -> Vector Concatenate/2
  Vector Concatenate/1 -> MatrixMultiply/2
  Constant/1 -> MatrixMultiply/1
  Constant1/1 -> MatrixMultiply1/1
  Constant2/1 -> MatrixMultiply2/1
  Constant3/1 -> MatrixMultiply3/1
  MatrixMultiply/1 -> Sum of Elements/1
  MatrixMultiply1/1 -> Sum of Elements/2
  MatrixMultiply2/1 -> Sum of Elements/3
  MatrixMultiply3/1 -> Sum of Elements/4
  Sum of Elements/1 -> Demux/1
  Demux/1 -> Out1/1
  Demux/2 -> Out2/1
  In4/1 -> Vector Concatenate1/2
  In5/1 -> Vector Concatenate2/1
  In6/1 -> Vector Concatenate2/2
  In7/1 -> Vector Concatenate3/1
  In8/1 -> Vector Concatenate3/2
  Vector Concatenate1/1 -> MatrixMultiply1/2
  Vector Concatenate2/1 -> MatrixMultiply2/2
  Vector Concatenate3/1 -> MatrixMultiply3/2
  In3/1 -> Vector Concatenate1/1

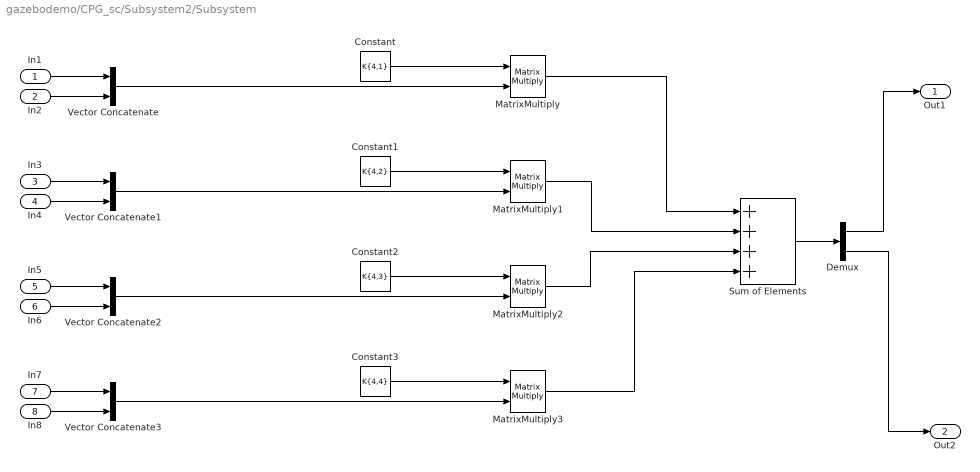
== system gazebodemo/CPG_sc/Subsystem2/Subsystem ==
  In1 : Inport
  In2 : Inport  Port=2
  In3 : Inport  Port=3
  In4 : Inport  Port=4
  In5 : Inport  Port=5
  In6 : Inport  Port=6
  In7 : Inport  Port=7
  In8 : Inport  Port=8
  Constant : Constant  Value=K{4,1}  VectorParams1D=off
  Constant1 : Constant  Value=K{4,2}  VectorParams1D=off
  Constant2 : Constant  Value=K{4,3}  VectorParams1D=off
  Constant3 : Constant  Value=K{4,4}  VectorParams1D=off
  Demux : Demux  Outputs=2
  MatrixMultiply{,1..3} (4 alike) : Product  Multiplication=Matrix(*)
  Sum of Elements : Sum  Inputs=++++
  Vector Concatenate{,1..3} (4 alike) : Concatenate
  Out1 : Outport
  Out2 : Outport  Port=2
  wires:
  In1/1 -> Vector Concatenate/1
  In2/1 -> Vector Concatenate/2
  Vector Concatenate/1 -> MatrixMultiply/2
  Constant/1 -> MatrixMultiply/1
  Constant1/1 -> MatrixMultiply1/1
  Constant2/1 -> MatrixMultiply2/1
  Constant3/1 -> MatrixMultiply3/1
  MatrixMultiply/1 -> Sum of Elements/1
  MatrixMultiply1/1 -> Sum of Elements/2
  MatrixMultiply2/1 -> Sum of Elements/3
  MatrixMultiply3/1 -> Sum of Elements/4
  Sum of Elements/1 -> Demux/1
  Demux/1 -> Out1/1
  Demux/2 -> Out2/1
  In4/1 -> Vector Concatenate1/2
  In5/1 -> Vector Concatenate2/1
  In6/1 -> Vector Concatenate2/2
  In7/1 -> Vector Concatenate3/1
  In8/1 -> Vector Concatenate3/2
  Vector Concatenate1/1 -> MatrixMultiply1/2
  Vector Concatenate2/1 -> MatrixMultiply2/2
  Vector Concatenate3/1 -> MatrixMultiply3/2
  In3/1 -> Vector Concatenate1/1

== system gazebodemo/Subsystem/nonlinear compensation/Coriolis + centrifugal ==
  q : Inport
  dq : Inport  Port=2
  Demux2 : Demux  Outputs=2
      settings: DisplayOption=none
  Fcn1 : Fcn  Expr=sin(u(2))  SampleTime=Tc
  Gain : Gain  Gain=-a(1)*pi_m(3)  SaturateOnIntegerOverflow=on  OutDataTypeStr=Inherit: Same as input  ParamDataTypeStr=Inherit: Same as input
      mask Display: disp('k_3')
  Gain1 : Gain  Gain=2  SaturateOnIntegerOverflow=on  OutDataTypeStr=Inherit: Same as input  ParamDataTypeStr=Inherit: Same as input
  Gain2 : Gain  Gain=-1  SaturateOnIntegerOverflow=on  OutDataTypeStr=Inherit: Same as input  ParamDataTypeStr=Inherit: Same as input
  Mux : Mux  Inputs=2
  Product{4..7} (4 alike) : Product  InputSameDT=on  RndMeth=Zero  SaturateOnIntegerOverflow=on  SampleTime=Tc  OutDataTypeStr=Inherit: Same as first input
  Sum : Sum  InputSameDT=on  SaturateOnIntegerOverflow=on  OutDataTypeStr=Inherit: Same as first input
  prdiuct 1 : Product  InputSameDT=on  RndMeth=Zero  SaturateOnIntegerOverflow=on  SampleTime=Tc  OutDataTypeStr=Inherit: Same as first input
  Cdq : Outport  InitialOutput=0
  wires:
  Demux2/2 -> Product5/2, Product4/2
  dq/1 -> Demux2/1
  q/1 -> Fcn1/1
  Gain2/1 -> Mux/2
  Product6/1 -> Gain2/1
  Mux/1 -> Cdq/1
  Sum/1 -> Mux/1
  Product5/1 -> Sum/2
  Gain1/1 -> Sum/1
  Product7/1 -> Gain1/1
  prdiuct 1/1 -> Product6/1
  Gain/1 -> Product4/1, prdiuct 1/1
  Fcn1/1 -> Gain/1
  Demux2/1 -> Product7/1, Product6/2, prdiuct 1/2
  Product4/1 -> Product7/2, Product5/1

== system gazebodemo/Subsystem/nonlinear compensation/gravity ==
  q : Inport
  Demux : Demux  Outputs=2
      settings: DisplayOption=none
  Fcn1 : Fcn  Expr=cos(u)  SampleTime=Tc
  Fcn2 : Fcn  Expr=cos(u)  SampleTime=Tc
  Gain : Gain  Gain=g*pi_m(3)  SaturateOnIntegerOverflow=on  OutDataTypeStr=Inherit: Same as input  ParamDataTypeStr=Inherit: Same as input
      mask Display: disp('k_2')
  Gain1 : Gain  Gain=g*pi_m(1)  SaturateOnIntegerOverflow=on  OutDataTypeStr=Inherit: Same as input  ParamDataTypeStr=Inherit: Same as input
      mask Display: disp('k_1')
  Mux : Mux  Inputs=2
  Sum2 : Sum  InputSameDT=on  SaturateOnIntegerOverflow=on  SampleTime=Tc  OutDataTypeStr=Inherit: Same as first input
  Sum5 : Sum  InputSameDT=on  SaturateOnIntegerOverflow=on  OutDataTypeStr=Inherit: Same as first input
  g : Outport  InitialOutput=0
  wires:
  Mux/1 -> g/1
  Gain/1 -> Sum5/2, Mux/2
  Sum5/1 -> Mux/1
  Gain1/1 -> Sum5/1
  Demux/1 -> Sum2/1, Fcn2/1
  Fcn2/1 -> Gain1/1
  Fcn1/1 -> Gain/1
  Sum2/1 -> Fcn1/1
  Demux/2 -> Sum2/2
  q/1 -> Demux/1

== system gazebodemo/Subsystem1/nonlinear compensation/Coriolis + centrifugal ==
  q : Inport
  dq : Inport  Port=2
  Demux2 : Demux  Outputs=2
      settings: DisplayOption=none
  Fcn1 : Fcn  Expr=sin(u(2))  SampleTime=Tc
  Gain : Gain  Gain=-a(1)*pi_m(3)  SaturateOnIntegerOverflow=on  OutDataTypeStr=Inherit: Same as input  ParamDataTypeStr=Inherit: Same as input
      mask Display: disp('k_3')
  Gain1 : Gain  Gain=2  SaturateOnIntegerOverflow=on  OutDataTypeStr=Inherit: Same as input  ParamDataTypeStr=Inherit: Same as input
  Gain2 : Gain  Gain=-1  SaturateOnIntegerOverflow=on  OutDataTypeStr=Inherit: Same as input  ParamDataTypeStr=Inherit: Same as input
  Mux : Mux  Inputs=2
  Product{4..7} (4 alike) : Product  InputSameDT=on  RndMeth=Zero  SaturateOnIntegerOverflow=on  SampleTime=Tc  OutDataTypeStr=Inherit: Same as first input
  Sum : Sum  InputSameDT=on  SaturateOnIntegerOverflow=on  OutDataTypeStr=Inherit: Same as first input
  prdiuct 1 : Product  InputSameDT=on  RndMeth=Zero  SaturateOnIntegerOverflow=on  SampleTime=Tc  OutDataTypeStr=Inherit: Same as first input
  Cdq : Outport  InitialOutput=0
  wires:
  Demux2/2 -> Product5/2, Product4/2
  dq/1 -> Demux2/1
  q/1 -> Fcn1/1
  Gain2/1 -> Mux/2
  Product6/1 -> Gain2/1
  Mux/1 -> Cdq/1
  Sum/1 -> Mux/1
  Product5/1 -> Sum/2
  Gain1/1 -> Sum/1
  Product7/1 -> Gain1/1
  prdiuct 1/1 -> Product6/1
  Gain/1 -> Product4/1, prdiuct 1/1
  Fcn1/1 -> Gain/1
  Demux2/1 -> Product7/1, Product6/2, prdiuct 1/2
  Product4/1 -> Product7/2, Product5/1

== system gazebodemo/Subsystem1/nonlinear compensation/gravity ==
  q : Inport
  Demux : Demux  Outputs=2
      settings: DisplayOption=none
  Fcn1 : Fcn  Expr=cos(u)  SampleTime=Tc
  Fcn2 : Fcn  Expr=cos(u)  SampleTime=Tc
  Gain : Gain  Gain=g*pi_m(3)  SaturateOnIntegerOverflow=on  OutDataTypeStr=Inherit: Same as input  ParamDataTypeStr=Inherit: Same as input
      mask Display: disp('k_2')
  Gain1 : Gain  Gain=g*pi_m(1)  SaturateOnIntegerOverflow=on  OutDataTypeStr=Inherit: Same as input  ParamDataTypeStr=Inherit: Same as input
      mask Display: disp('k_1')
  Mux : Mux  Inputs=2
  Sum2 : Sum  InputSameDT=on  SaturateOnIntegerOverflow=on  SampleTime=Tc  OutDataTypeStr=Inherit: Same as first input
  Sum5 : Sum  InputSameDT=on  SaturateOnIntegerOverflow=on  OutDataTypeStr=Inherit: Same as first input
  g : Outport  InitialOutput=0
  wires:
  Mux/1 -> g/1
  Gain/1 -> Sum5/2, Mux/2
  Sum5/1 -> Mux/1
  Gain1/1 -> Sum5/1
  Demux/1 -> Sum2/1, Fcn2/1
  Fcn2/1 -> Gain1/1
  Fcn1/1 -> Gain/1
  Sum2/1 -> Fcn1/1
  Demux/2 -> Sum2/2
  q/1 -> Demux/1

== system gazebodemo/Subsystem2/nonlinear compensation/Coriolis + centrifugal ==
  q : Inport
  dq : Inport  Port=2
  Demux2 : Demux  Outputs=2
      settings: DisplayOption=none
  Fcn1 : Fcn  Expr=sin(u(2))  SampleTime=Tc
  Gain : Gain  Gain=-a(1)*pi_m(3)  SaturateOnIntegerOverflow=on  OutDataTypeStr=Inherit: Same as input  ParamDataTypeStr=Inherit: Same as input
      mask Display: disp('k_3')
  Gain1 : Gain  Gain=2  SaturateOnIntegerOverflow=on  OutDataTypeStr=Inherit: Same as input  ParamDataTypeStr=Inherit: Same as input
  Gain2 : Gain  Gain=-1  SaturateOnIntegerOverflow=on  OutDataTypeStr=Inherit: Same as input  ParamDataTypeStr=Inherit: Same as input
  Mux : Mux  Inputs=2
  Product{4..7} (4 alike) : Product  InputSameDT=on  RndMeth=Zero  SaturateOnIntegerOverflow=on  SampleTime=Tc  OutDataTypeStr=Inherit: Same as first input
  Sum : Sum  InputSameDT=on  SaturateOnIntegerOverflow=on  OutDataTypeStr=Inherit: Same as first input
  prdiuct 1 : Product  InputSameDT=on  RndMeth=Zero  SaturateOnIntegerOverflow=on  SampleTime=Tc  OutDataTypeStr=Inherit: Same as first input
  Cdq : Outport  InitialOutput=0
  wires:
  Demux2/2 -> Product5/2, Product4/2
  dq/1 -> Demux2/1
  q/1 -> Fcn1/1
  Gain2/1 -> Mux/2
  Product6/1 -> Gain2/1
  Mux/1 -> Cdq/1
  Sum/1 -> Mux/1
  Product5/1 -> Sum/2
  Gain1/1 -> Sum/1
  Product7/1 -> Gain1/1
  prdiuct 1/1 -> Product6/1
  Gain/1 -> Product4/1, prdiuct 1/1
  Fcn1/1 -> Gain/1
  Demux2/1 -> Product7/1, Product6/2, prdiuct 1/2
  Product4/1 -> Product7/2, Product5/1

== system gazebodemo/Subsystem2/nonlinear compensation/gravity ==
  q : Inport
  Demux : Demux  Outputs=2
      settings: DisplayOption=none
  Fcn1 : Fcn  Expr=cos(u)  SampleTime=Tc
  Fcn2 : Fcn  Expr=cos(u)  SampleTime=Tc
  Gain : Gain  Gain=g*pi_m(3)  SaturateOnIntegerOverflow=on  OutDataTypeStr=Inherit: Same as input  ParamDataTypeStr=Inherit: Same as input
      mask Display: disp('k_2')
  Gain1 : Gain  Gain=g*pi_m(1)  SaturateOnIntegerOverflow=on  OutDataTypeStr=Inherit: Same as input  ParamDataTypeStr=Inherit: Same as input
      mask Display: disp('k_1')
  Mux : Mux  Inputs=2
  Sum2 : Sum  InputSameDT=on  SaturateOnIntegerOverflow=on  SampleTime=Tc  OutDataTypeStr=Inherit: Same as first input
  Sum5 : Sum  InputSameDT=on  SaturateOnIntegerOverflow=on  OutDataTypeStr=Inherit: Same as first input
  g : Outport  InitialOutput=0
  wires:
  Mux/1 -> g/1
  Gain/1 -> Sum5/2, Mux/2
  Sum5/1 -> Mux/1
  Gain1/1 -> Sum5/1
  Demux/1 -> Sum2/1, Fcn2/1
  Fcn2/1 -> Gain1/1
  Fcn1/1 -> Gain/1
  Sum2/1 -> Fcn1/1
  Demux/2 -> Sum2/2
  q/1 -> Demux/1

== system gazebodemo/Subsystem3/nonlinear compensation/Coriolis + centrifugal ==
  q : Inport
  dq : Inport  Port=2
  Demux2 : Demux  Outputs=2
      settings: DisplayOption=none
  Fcn1 : Fcn  Expr=sin(u(2))  SampleTime=Tc
  Gain : Gain  Gain=-a(1)*pi_m(3)  SaturateOnIntegerOverflow=on  OutDataTypeStr=Inherit: Same as input  ParamDataTypeStr=Inherit: Same as input
      mask Display: disp('k_3')
  Gain1 : Gain  Gain=2  SaturateOnIntegerOverflow=on  OutDataTypeStr=Inherit: Same as input  ParamDataTypeStr=Inherit: Same as input
  Gain2 : Gain  Gain=-1  SaturateOnIntegerOverflow=on  OutDataTypeStr=Inherit: Same as input  ParamDataTypeStr=Inherit: Same as input
  Mux : Mux  Inputs=2
  Product{4..7} (4 alike) : Product  InputSameDT=on  RndMeth=Zero  SaturateOnIntegerOverflow=on  SampleTime=Tc  OutDataTypeStr=Inherit: Same as first input
  Sum : Sum  InputSameDT=on  SaturateOnIntegerOverflow=on  OutDataTypeStr=Inherit: Same as first input
  prdiuct 1 : Product  InputSameDT=on  RndMeth=Zero  SaturateOnIntegerOverflow=on  SampleTime=Tc  OutDataTypeStr=Inherit: Same as first input
  Cdq : Outport  InitialOutput=0
  wires:
  Demux2/2 -> Product5/2, Product4/2
  dq/1 -> Demux2/1
  q/1 -> Fcn1/1
  Gain2/1 -> Mux/2
  Product6/1 -> Gain2/1
  Mux/1 -> Cdq/1
  Sum/1 -> Mux/1
  Product5/1 -> Sum/2
  Gain1/1 -> Sum/1
  Product7/1 -> Gain1/1
  prdiuct 1/1 -> Product6/1
  Gain/1 -> Product4/1, prdiuct 1/1
  Fcn1/1 -> Gain/1
  Demux2/1 -> Product7/1, Product6/2, prdiuct 1/2
  Product4/1 -> Product7/2, Product5/1

== system gazebodemo/Subsystem3/nonlinear compensation/gravity ==
  q : Inport
  Demux : Demux  Outputs=2
      settings: DisplayOption=none
  Fcn1 : Fcn  Expr=cos(u)  SampleTime=Tc
  Fcn2 : Fcn  Expr=cos(u)  SampleTime=Tc
  Gain : Gain  Gain=g*pi_m(3)  SaturateOnIntegerOverflow=on  OutDataTypeStr=Inherit: Same as input  ParamDataTypeStr=Inherit: Same as input
      mask Display: disp('k_2')
  Gain1 : Gain  Gain=g*pi_m(1)  SaturateOnIntegerOverflow=on  OutDataTypeStr=Inherit: Same as input  ParamDataTypeStr=Inherit: Same as input
      mask Display: disp('k_1')
  Mux : Mux  Inputs=2
  Sum2 : Sum  InputSameDT=on  SaturateOnIntegerOverflow=on  SampleTime=Tc  OutDataTypeStr=Inherit: Same as first input
  Sum5 : Sum  InputSameDT=on  SaturateOnIntegerOverflow=on  OutDataTypeStr=Inherit: Same as first input
  g : Outport  InitialOutput=0
  wires:
  Mux/1 -> g/1
  Gain/1 -> Sum5/2, Mux/2
  Sum5/1 -> Mux/1
  Gain1/1 -> Sum5/1
  Demux/1 -> Sum2/1, Fcn2/1
  Fcn2/1 -> Gain1/1
  Fcn1/1 -> Gain/1
  Sum2/1 -> Fcn1/1
  Demux/2 -> Sum2/2
  q/1 -> Demux/1
